simulink model "FINAL_CHBSPWM_9level_Fixed_DC_2"  (R2014a)
settings: Solver=ode45  StartTime=0.0  StopTime=0.4  RelTol=1e-3
libraries: powerlib x32, simulink x8
settings Model: Creator=KOUSIK  LastModifiedBy=PRAKASH BABU

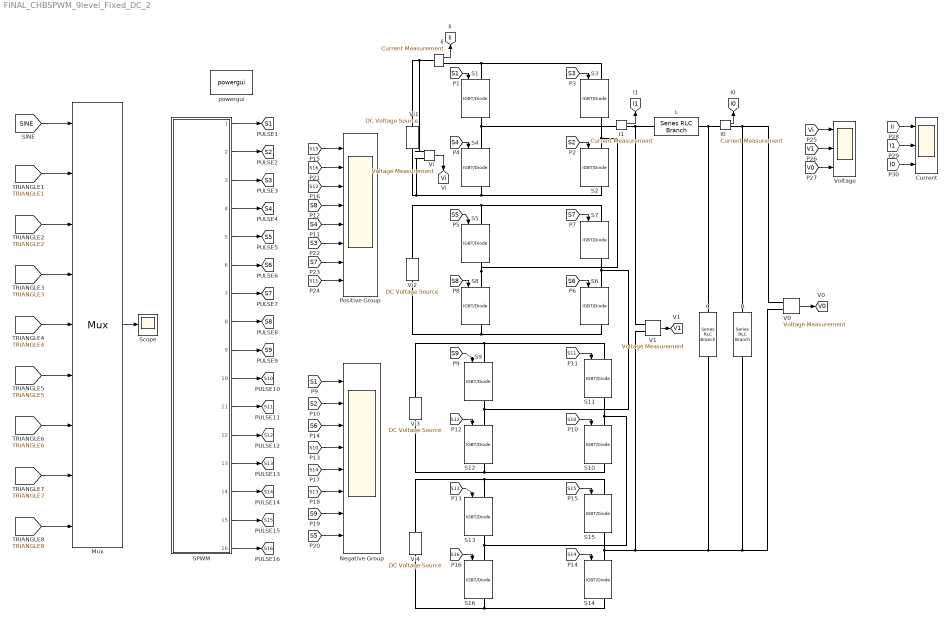
== system FINAL_CHBSPWM_9level_Fixed_DC_2 ==
  C : powerlib/Elements/Series RLC Branch  LConnTagsString=__new0  RConnTagsString=__new0  BranchType=C  Resistance=20  Inductance=5e-3  SetiL0=off  InitialCurrent=0  Capacitance=3.5e-6  Setx0=off  InitialVoltage=0  Measurements=None
  Current : Scope  NumInputPorts=3
      settings: TimeRange=0.1  YMin=-2~-5~-5  YMax=5~5~5  SaveName=current
  I0 : powerlib/Measurements/Current Measurement  PhasorSimulation=off  OutputType=Complex  PSBequivalent=0
  I1 : powerlib/Measurements/Current Measurement  PhasorSimulation=off  OutputType=Complex  PSBequivalent=0
  Ii : powerlib/Measurements/Current Measurement  PhasorSimulation=off  OutputType=Complex  PSBequivalent=0
  L : powerlib/Elements/Series RLC Branch  LConnTagsString=__new0  RConnTagsString=__new0  BranchType=L  Resistance=20  Inductance=20e-3  SetiL0=off  InitialCurrent=0  Capacitance=1e-6  Setx0=off  InitialVoltage=0  Measurements=None
  Mux : Mux  Inputs=9
  Negative Group : Scope  NumInputPorts=8
      settings: YMin=-5~-5~-5~-5~-5~-5~-5~-5  YMax=5~5~5~5~5~5~5~5  SaveName=negative
  Positive Group : Scope  NumInputPorts=8
      settings: YMin=-5~-5~-5~-5~-5~-5~-5~-5  YMax=5~5~5~5~5~5~5~5  SaveName=positive
  R : powerlib/Elements/Series RLC Branch  LConnTagsString=__new0  RConnTagsString=__new0  BranchType=R  Resistance=90  Inductance=5e-3  SetiL0=off  InitialCurrent=0  Capacitance=1e-6  Setx0=off  InitialVoltage=0  Measurements=None
  S{1..16} (16 alike) : powerlib/Power Electronics/IGBT//Diode  Ron=1e-3  Rs=1e5  Cs=inf  Measurements=on
  SPWM : Subsystem
  Scope : Scope
      settings: TickLabels=on  SaveName=sine
  "V0  " : powerlib/Measurements/Voltage Measurement  PhasorSimulation=off  OutputType=Complex  PSBequivalent=0
  "V1  " : powerlib/Measurements/Voltage Measurement  PhasorSimulation=off  OutputType=Complex  PSBequivalent=0
  Vi : powerlib/Measurements/Voltage Measurement  PhasorSimulation=off  OutputType=Complex  PSBequivalent=0
  Vi{1..4} (4 alike) : powerlib/Electrical Sources/DC Voltage Source  Amplitude=57.5  Measurements=None
  Voltage : Scope  NumInputPorts=3
      settings: TimeRange=0.1  YMin=56.5~-300~-300  YMax=58.5~300~300  SaveName=voltage
  powergui : powerlib/powergui  Priority=1  SimulationMode=Discrete  SolverType=Tustin  SampleTime=50e-6  frequency=60  SPID=off  DisableSnubberDevices=off  DisableRonSwitches=off  DisableVfSwitches=off  SwTol=0  Interpol=off  DisplayEquations=off  Ts=0  methode=off  frequencyindice=0  Pbase=100e6  ErrMax=1e-4  Iterations=50  UnitsV=kV  UnitsW=MW  FunctionMessages=off  echomessages=off  HookPort=off  EnableUseOfTLC=off  x0status=blocks  RestoreLinks=warning  ResistiveCurrentMeasurement=off  Frange=[0:2:500]  Ylog=off  Xlog=on  ShowGrid=off  save=off  variable=ZData  structure=voltage  ZoomFFT=off  StartTime=0.02  cycles=1  DisplayStyle=3  fundamental=50  FreqAxis=off  MaxFrequency=1000  frequencyindicesteady=1  RmsSteady=1  display=off
  tag scope: I0=global, I1=global, Ii=global, S10=global, S11=global, S12=global, S13=global, S14=global, S15=global, S16=global, S1=global, S2=global, S3=global, S4=global, S5=global, S6=global, S7=global, S8=global, S9=global, V0=global, V1=global, Vi=global
  wires:
  [SINE] -> Mux/1
  [TRIANGLE1] -> Mux/2
  [TRIANGLE2] -> Mux/3
  [TRIANGLE3] -> Mux/4
  [TRIANGLE4] -> Mux/5
  Mux/1 -> Scope/1
  [S1] -> S1/1
  [S2] -> S2/1
  [S3] -> S3/1
  [S4] -> S4/1
  [S5] -> S5/1
  [S6] -> S6/1
  [S7] -> S7/1
  [S8] -> S8/1
  [S1] -> Negative Group/1
  [S2] -> Negative Group/2
  [S6] -> Negative Group/3
  [S10] -> Negative Group/4
  [S15] -> Positive Group/1
  [S16] -> Positive Group/2
  [S12] -> Positive Group/3
  [S8] -> Positive Group/4
  [S9] -> S9/1
  [S10] -> S10/1
  [S11] -> S11/1
  [S12] -> S12/1
  [S13] -> S13/1
  [S14] -> S14/1
  [S15] -> S15/1
  [S16] -> S16/1
  [TRIANGLE5] -> Mux/6
  [TRIANGLE6] -> Mux/7
  [TRIANGLE7] -> Mux/8
  [TRIANGLE8] -> Mux/9
  [S14] -> Negative Group/5
  [S13] -> Negative Group/6
  [S9] -> Negative Group/7
  [S5] -> Negative Group/8
  [S4] -> Positive Group/5
  [S3] -> Positive Group/6
  [S7] -> Positive Group/7
  [S11] -> Positive Group/8
  SPWM/1(1) -> [S1]
  "V0  "/1 -> [V0]
  "V1  "/1 -> [V1]
  Vi/1 -> [Vi]
  Ii/1 -> [Ii]
  I1/1 -> [I1]
  I0/1 -> [I0]
  [V0] -> Voltage/3
  [V1] -> Voltage/2
  [Vi] -> Voltage/1
  [I0] -> Current/3
  [I1] -> Current/2
  [Ii] -> Current/1
  SPWM/16(16) -> [S16]
  SPWM/15(15) -> [S15]
  SPWM/14(14) -> [S14]
  SPWM/13(13) -> [S13]
  SPWM/12(12) -> [S12]
  SPWM/11(11) -> [S11]
  SPWM/10(10) -> [S10]
  SPWM/9(9) -> [S9]
  SPWM/2(2) -> [S2]
  SPWM/3(3) -> [S3]
  SPWM/4(4) -> [S4]
  SPWM/5(5) -> [S5]
  SPWM/6(6) -> [S6]
  SPWM/7(7) -> [S7]
  SPWM/8(8) -> [S8]
  connections:
  Vi/LConn1 -- Vi1/RConn1 -- Ii/LConn1
  S4/RConn1 -- Vi1/LConn1 -- Vi/LConn2 -- S2/RConn1
  "V1  "/LConn1 -- I1/RConn1 -- L/RConn1
  S7/LConn1 -- S5/LConn1 -- Vi2/RConn1
  Vi2/LConn1 -- S8/RConn1 -- S6/RConn1
  S2/LConn1 -- S3/RConn1 -- S8/LConn1 -- S5/RConn1
  S11/LConn1 -- Vi3/RConn1 -- S9/LConn1
  Vi3/LConn1 -- S10/RConn1 -- S12/RConn1
  S6/LConn1 -- S12/LConn1 -- S9/RConn1 -- S7/RConn1
  Vi4/RConn1 -- S15/LConn1 -- S13/LConn1
  S14/RConn1 -- Vi4/LConn1 -- S16/RConn1
  S10/LConn1 -- S16/LConn1 -- S13/RConn1 -- S11/RConn1
  S14/LConn1 -- C/RConn1 -- "V0  "/LConn2 -- R/RConn1 -- "V1  "/LConn2 -- S15/RConn1
  C/LConn1 -- I0/LConn1 -- L/LConn1
  S1/LConn1 -- Ii/RConn1 -- S3/LConn1
  S4/LConn1 -- I1/LConn1 -- S1/RConn1
  R/LConn1 -- I0/RConn1 -- "V0  "/LConn1

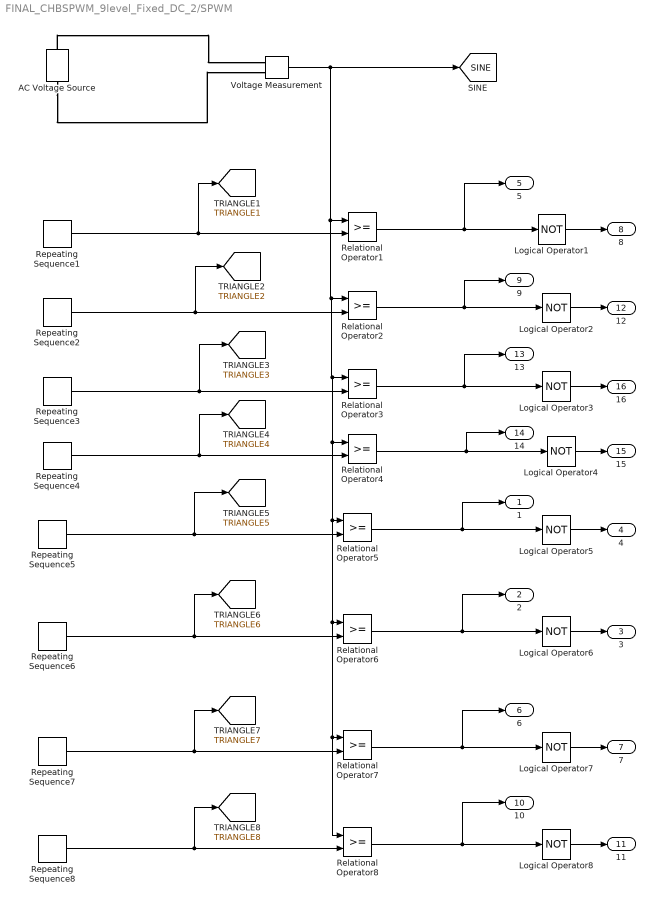
== system FINAL_CHBSPWM_9level_Fixed_DC_2/SPWM ==
  AC Voltage Source : powerlib/Electrical Sources/AC Voltage Source  Amplitude=4  Phase=0  Frequency=50  SampleTime=0  Measurements=None
  Logical Operator{1..8} (8 alike) : Logic  Operator=NOT  AllPortsSameDT=off  OutDataTypeStr=boolean
  Relational Operator{1..8} (8 alike) : RelationalOperator  OutDataTypeStr=boolean
  Repeating Sequence1 : simulink/Sources/Repeating Sequence  rep_seq_t=[0 0.5 1]/2500  rep_seq_y=[3 4 3]
  Repeating Sequence2 : simulink/Sources/Repeating Sequence  rep_seq_t=[0 0.5 1]/2500  rep_seq_y=[2 3 2]
  Repeating Sequence3 : simulink/Sources/Repeating Sequence  rep_seq_t=[0 0.5 1]/2500  rep_seq_y=[1 2 1]
  Repeating Sequence4 : simulink/Sources/Repeating Sequence  rep_seq_t=[0 0.5 1]/2500  rep_seq_y=[0 1 0]
  Repeating Sequence5 : simulink/Sources/Repeating Sequence  rep_seq_t=[0 0.5 1]/2500  rep_seq_y=[-1 0 -1]
  Repeating Sequence6 : simulink/Sources/Repeating Sequence  rep_seq_t=[0 0.5 1]/2500  rep_seq_y=[-2 -1 -2]
  Repeating Sequence7 : simulink/Sources/Repeating Sequence  rep_seq_t=[0 0.5 1]/2500  rep_seq_y=[-3 -2 -3]
  Repeating Sequence8 : simulink/Sources/Repeating Sequence  rep_seq_t=[0 0.5 1]/2500  rep_seq_y=[-4 -3 -4]
  Voltage Measurement : powerlib/Measurements/Voltage Measurement  PhasorSimulation=off  OutputType=Complex  PSBequivalent=0
  1 : Outport
  2 : Outport  Port=2
  3 : Outport  Port=3
  4 : Outport  Port=4
  5 : Outport  Port=5
  6 : Outport  Port=6
  7 : Outport  Port=7
  8 : Outport  Port=8
  9 : Outport  Port=9
  10 : Outport  Port=10
  11 : Outport  Port=11
  12 : Outport  Port=12
  13 : Outport  Port=13
  14 : Outport  Port=14
  15 : Outport  Port=15
  16 : Outport  Port=16
  tag scope: SINE=global, TRIANGLE1=global, TRIANGLE2=global, TRIANGLE3=global, TRIANGLE4=global, TRIANGLE5=global, TRIANGLE6=global, TRIANGLE7=global, TRIANGLE8=global
  wires:
  Logical Operator1/1 -> 8/1
  Relational Operator1/1 -> 5/1, Logical Operator1/1
  Repeating Sequence2/1 -> [TRIANGLE2], Relational Operator2/2
  Relational Operator2/1 -> 9/1, Logical Operator2/1
  Voltage Measurement/1 -> Relational Operator4/1, Relational Operator6/1, Relational Operator7/1, Relational Operator8/1, Relational Operator5/1, Relational Operator3/1, Relational Operator2/1, Relational Operator1/1, [SINE]
  Relational Operator3/1 -> 13/1, Logical Operator3/1
  Repeating Sequence1/1 -> [TRIANGLE1], Relational Operator1/2
  Repeating Sequence3/1 -> [TRIANGLE3], Relational Operator3/2
  Logical Operator2/1 -> 12/1
  Relational Operator4/1 -> 14/1, Logical Operator4/1
  Repeating Sequence4/1 -> [TRIANGLE4], Relational Operator4/2
  Logical Operator3/1 -> 16/1
  Logical Operator4/1 -> 15/1
  Repeating Sequence5/1 -> [TRIANGLE5], Relational Operator5/2
  Logical Operator5/1 -> 4/1
  Relational Operator6/1 -> 2/1, Logical Operator6/1
  Repeating Sequence6/1 -> [TRIANGLE6], Relational Operator6/2
  Logical Operator6/1 -> 3/1
  Relational Operator7/1 -> 6/1, Logical Operator7/1
  Repeating Sequence7/1 -> [TRIANGLE7], Relational Operator7/2
  Logical Operator7/1 -> 7/1
  Relational Operator8/1 -> 10/1, Logical Operator8/1
  Repeating Sequence8/1 -> [TRIANGLE8], Relational Operator8/2
  Logical Operator8/1 -> 11/1
  Relational Operator5/1 -> 1/1, Logical Operator5/1
  connections:
  AC Voltage Source/LConn1 -- Voltage Measurement/LConn2
  AC Voltage Source/RConn1 -- Voltage Measurement/LConn1
